simulink model "SimpleBot_V2"  (R2024a)
settings: Solver=VariableStepAuto  StartTime=0.0  StopTime=10  RelTol=1e-3
PreLoadFcn:
  | run('Parameter.m')
values from neighbouring files (symbols this model uses):
  Achsabstand = 0.15    [Model1Sensibilities.m]    (also in Model1numericalPSA.m; Model2Sensibilities.m; Modellvalidierung.m; MotorSens2.m)
  Reifen_Radius = 0.04    [Model1Sensibilities.m]    (also in Model1numericalPSA.m; Model2Sensibilities.m; Modellvalidierung.m; MotorSens2.m)
settings Model: Creator=jakob  LastModifiedBy=jakob

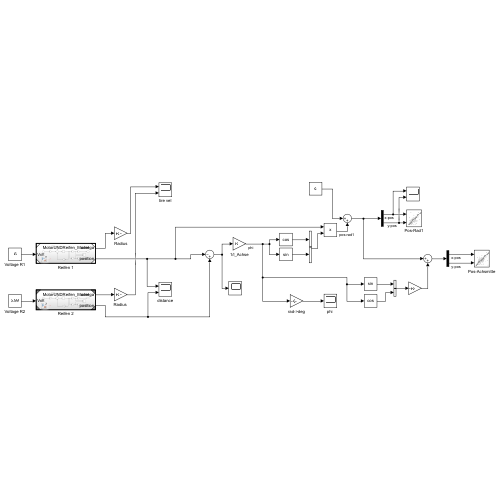
[thumbnail: Simulink's stored preview of the top-level diagram]
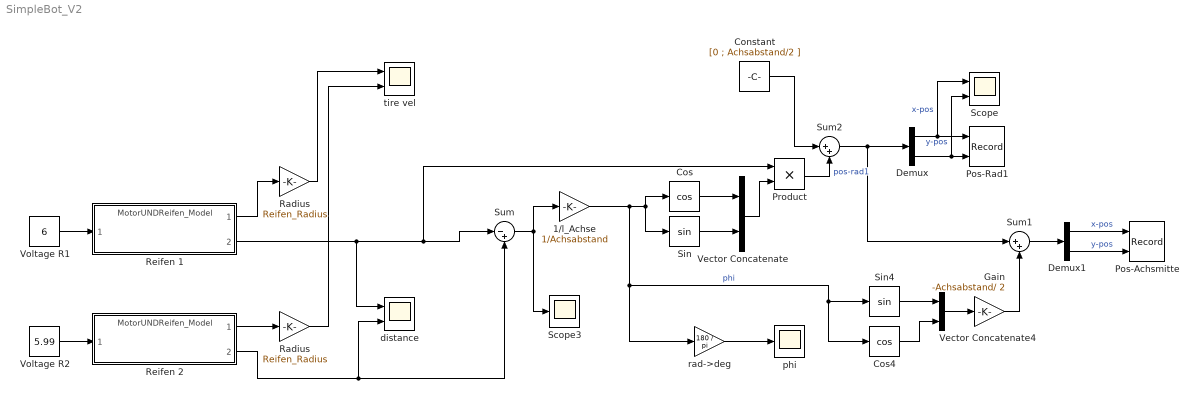
== system SimpleBot_V2 ==
  1/l_Achse : Gain  Gain=1/Achsabstand
  Constant : Constant  Value=[0 ; Achsabstand/2 ]
  Cos : Trigonometry  Operator=cos
  Cos4 : Trigonometry  Operator=cos
  Demux : Demux  Outputs=2
  Demux1 : Demux  Outputs=2
  Gain : Gain  Gain=-Achsabstand/ 2
  Pos-Achsmitte : Record  FileSettingsInternal="{\"entries\":[{\"content\":{\"excelSettings\":{\"content\":{},\"type\":\"Streamout.ExcelSettings\"}},\"type\":\"Streamout.FileSettingStorage\",\"uuid\":\"\"}],\"packageUris\":[\"http:\\/\\/schema.mathworks.com\\/mf0\\/streamout_blocks\\/R2020a\"],\"version\":\"1.0\"}"  Layout=[1 1]  SignalsInternal="{\"entries\":[{\"content\":{\"signals\":[{\"content\":{\"blockPath\":[],\"dimensions\":[1],\"domain\":\"\",\"lineColor\":\"#fe330a\",\"lineWidth\":2,\"plots\":[ 1 ],\"port\":1,\"signalID\":1,\"signalName\":\"x-pos\"},\"type\":\"RecordBlkView.Signal\",\"uuid\":\"\"},{\"content\":{\"blockPath\":[],\"dimensions\":[1],\"domain\":\"\",\"lineColor\":\"#22b573\",\"lineWidth\":2,\"plots\":[ 1 ],\"port\":2,\"signalID\":2,\"signalName\":\"y-pos\"},\"type\":\"RecordBlkView.Signal\",\"uuid\":\"\"}]},\"type\":\"RecordBlkView.InputSignals\",\"uuid\":\"\"}],\"packageUris\":[\"http:\\/\\/schema.mathworks.com\\/mf0\\/streamout_blocks\\/R2020a\"],\"version\":\"1.0\"}"  VisualizationBindings="{\"xyplotplugin\":{\"info\":[{\"series\":[{\"bindingParametersList\":[{\"parameter\":\"X-Axis\",\"signalID\":1,\"signalName\":\"x-pos\"},{\"parameter\":\"Y-Axis\",\"signalID\":2,\"signalName\":\"y-pos\"}],\"seriesID\":0}],\"subplotID\":1}]}}"  CompatibilityTag=XY  st=-1
  Pos-Rad1 : Record  FileSettingsInternal="{\"entries\":[{\"content\":{\"excelSettings\":{\"content\":{},\"type\":\"Streamout.ExcelSettings\"}},\"type\":\"Streamout.FileSettingStorage\",\"uuid\":\"\"}],\"packageUris\":[\"http:\\/\\/schema.mathworks.com\\/mf0\\/streamout_blocks\\/R2020a\"],\"version\":\"1.0\"}"  Layout=[1 1]  SignalsInternal="{\"entries\":[{\"content\":{\"signals\":[{\"content\":{\"blockPath\":[],\"dimensions\":[1],\"domain\":\"\",\"lineColor\":\"#0072bd\",\"lineWidth\":2,\"plots\":[ 1 ],\"port\":1,\"signalID\":1,\"signalName\":\"x-pos\"},\"type\":\"RecordBlkView.Signal\",\"uuid\":\"\"},{\"content\":{\"blockPath\":[],\"dimensions\":[1],\"domain\":\"\",\"lineColor\":\"#d95319\",\"lineWidth\":2,\"plots\":[ 1 ],\"port\":2,\"signalID\":2,\"signalName\":\"y-pos\"},\"type\":\"RecordBlkView.Signal\",\"uuid\":\"\"}]},\"type\":\"RecordBlkView.InputSignals\",\"uuid\":\"\"}],\"packageUris\":[\"http:\\/\\/schema.mathworks.com\\/mf0\\/streamout_blocks\\/R2020a\"],\"version\":\"1.0\"}"  VisualizationBindings="{\"xyplotplugin\":{\"info\":[{\"series\":[{\"bindingParametersList\":[{\"parameter\":\"X-Axis\",\"signalID\":1,\"signalName\":\"x-pos\"},{\"parameter\":\"Y-Axis\",\"signalID\":2,\"signalName\":\"y-pos\"}],\"seriesID\":0}],\"subplotID\":1}]}}"  CompatibilityTag=XY  st=-1
  Product : Product
  Radius : Gain  Gain=Reifen_Radius
  "Radius " : Gain  Gain=Reifen_Radius
  Reifen 1 : ModelReference  ModelNameDialog=MotorUNDReifen_Model.slx  SimulationMode=Normal  ModelReferenceVersion=1.5
  Reifen 2 : ModelReference  ModelNameDialog=MotorUNDReifen_Model.slx  SimulationMode=Normal  ModelReferenceVersion=1.5
  Scope : Scope  NumInputPorts=2
  Scope3 : Scope
  Sin : Trigonometry
  Sin4 : Trigonometry
  Sum : Sum  Inputs=|-+
  Sum1 : Sum  Inputs=|++
  Sum2 : Sum  Inputs=|++
  Vector Concatenate : Concatenate
  Vector Concatenate4 : Concatenate
  Voltage R1 : Constant  Value=6  SampleTime=4
  Voltage R2 : Constant  Value=5.99
  distance : Scope  NumInputPorts=2
  "phi " : Scope
  rad->deg : Gain  Gain=180 / pi
  tire vel : Scope  NumInputPorts=2
  wires:
  Voltage R1/1 -> Reifen 1/1
  Voltage R2/1 -> Reifen 2/1
  Reifen 1/1 -> Radius/1
  Reifen 2/1 -> "Radius "/1
  Reifen 1/2 -> distance/1, Sum/1, Product/1
  Sum1/1 -> Demux1/1
  Demux1/2 -> Pos-Achsmitte/2  "y-pos"
  Demux1/1 -> Pos-Achsmitte/1  "x-pos"
  Reifen 2/2 -> distance/2, Sum/2
  Gain/1 -> Sum1/2
  Cos4/1 -> Vector Concatenate4/2
  Demux/2 -> Scope/2, Pos-Rad1/2  "y-pos"
  Vector Concatenate4/1 -> Gain/1
  1/l_Achse/1 -> Sin/1, Cos/1, rad->deg/1, Cos4/1, Sin4/1  "phi"
  Cos/1 -> Vector Concatenate/1
  rad->deg/1 -> "phi "/1
  Vector Concatenate/1 -> Product/2
  Sum/1 -> 1/l_Achse/1, Scope3/1
  Demux/1 -> Scope/1, Pos-Rad1/1  "x-pos"
  Sin/1 -> Vector Concatenate/2
  Radius/1 -> tire vel/1
  "Radius "/1 -> tire vel/2
  Product/1 -> Sum2/2  "pos-rad1"
  Sum2/1 -> Sum1/1, Demux/1
  Constant/1 -> Sum2/1
  Sin4/1 -> Vector Concatenate4/1
